simulink model "FEAD_TestRig"  (R2026a)
settings: Solver=ode23t  StartTime=0  StopTime=30  MaxStep=1e-3  RelTol=1e-4  AbsTol=1e-6
libraries: fl_lib x41, nesl_utility x27, simulink x1
settings Model: Creator=RICARDO  LastModifiedBy=RICARDO

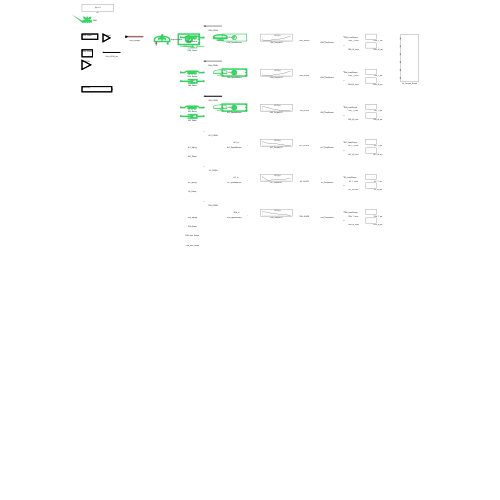
[thumbnail: Simulink's stored preview of the top-level diagram]
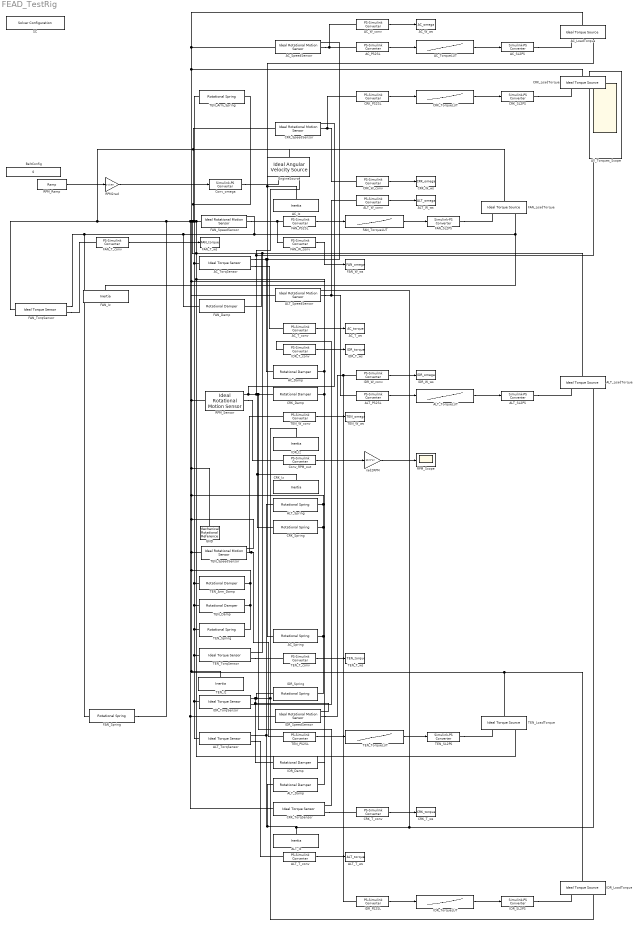
== system FEAD_TestRig ==
  AC_Damp : fl_lib/Mechanical/Rotational Elements/Rotational Damper  D=4.4060 N*m*s/rad  w_specify=off  w_priority=None  w=0 rad/s  w_nominal_specify=off  w_nominal_value=1  w_nominal_unit=rad/s  t_specify=off  t_priority=None  t=0 N*m  t_nominal_specify=off  t_nominal_value=1  t_nominal_unit=N*m
  AC_Iz : fl_lib/Mechanical/Rotational Elements/Inertia  inertia=0.005516 kg*m^2  num_ports=foundation.enum.numPorts2.one  w_specify=off  w_priority=High  w=0 rad/s  w_nominal_specify=off  w_nominal_value=1  w_nominal_unit=rad/s  t_specify=off  t_priority=None  t=0 N*m  t_nominal_specify=off  t_nominal_value=1  t_nominal_unit=N*m
  AC_LoadTorque : fl_lib/Mechanical/Mechanical Sources/Ideal Torque Source
  AC_PS2SL : nesl_utility/PS-Simulink Converter  PhysicalDomain=network_engine_domain  SubClassName=ps_output  LeftPortType=input  RightPortType=output  PseudoPeriodic=off  Frequencies=[]  VectorFormat=inherit  Unit=inherit  AffineConversion=off
  AC_SL2PS : nesl_utility/Simulink-PS Converter  PhysicalDomain=network_engine_domain  SubClassName=ps_input  LeftPortType=input  RightPortType=output  PseudoPeriodic=off  Frequencies=[]  NoiseDistribution=none  NoiseParameters=[]  Unit=1  AffineConversion=off  FilteringAndDerivatives=provide  SimscapeFilterOrder=1  InputFilterTimeConstant=0.001  UdotUserProvided=0
  AC_SpeedSensor : fl_lib/Mechanical/Mechanical Sensors/Ideal Rotational Motion Sensor  reference=foundation.enum.MeasurementReference.difference  acceleration_port=false  velocity_port=true  position_port=true  wrap_angle=false  offset=0 rad
  AC_Spring : fl_lib/Mechanical/Rotational Elements/Rotational Spring  spr_rate=4406.0 N*m/rad  w_specify=off  w_priority=None  w=0 rad/s  w_nominal_specify=off  w_nominal_value=1  w_nominal_unit=rad/s  t_specify=off  t_priority=None  t=0 N*m  t_nominal_specify=off  t_nominal_value=1  t_nominal_unit=N*m  phi_specify=off  phi_priority=High  phi=0 rad  phi_nominal_specify=off  phi_nominal_value=1  phi_nominal_unit=rad
  AC_T_conv : nesl_utility/PS-Simulink Converter  PhysicalDomain=network_engine_domain  SubClassName=ps_output  LeftPortType=input  RightPortType=output  PseudoPeriodic=off  Frequencies=[]  VectorFormat=inherit  Unit=inherit  AffineConversion=off
  AC_T_ws : ToWorkspace  VariableName=AC_torque  SampleTime=-1
  AC_TorqSensor : fl_lib/Mechanical/Mechanical Sensors/Ideal Torque Sensor
  AC_TorqueLUT : Lookup_n-D  NumberOfTableDimensions=1  BreakpointsForDimension1=[52.3599 83.7758 104.72 125.664 146.608 167.552 188.496 209.44]  Table=[19.0986 15.8757 16.5203 16.7113 16.5066 16.7113 17.4009 17.3797]  ExtrapMethod=Clip  InternalRulePriority=Speed  RndMeth=Simplest
  AC_W_conv : nesl_utility/PS-Simulink Converter  PhysicalDomain=network_engine_domain  SubClassName=ps_output  LeftPortType=input  RightPortType=output  PseudoPeriodic=off  Frequencies=[]  VectorFormat=inherit  Unit=inherit  AffineConversion=off
  AC_W_ws : ToWorkspace  VariableName=AC_omega  SampleTime=-1
  ALT_Damp : fl_lib/Mechanical/Rotational Elements/Rotational Damper  D=0.8823 N*m*s/rad  w_specify=off  w_priority=None  w=0 rad/s  w_nominal_specify=off  w_nominal_value=1  w_nominal_unit=rad/s  t_specify=off  t_priority=None  t=0 N*m  t_nominal_specify=off  t_nominal_value=1  t_nominal_unit=N*m
  ALT_Iz : fl_lib/Mechanical/Rotational Elements/Inertia  inertia=0.000543 kg*m^2  num_ports=foundation.enum.numPorts2.one  w_specify=off  w_priority=High  w=0 rad/s  w_nominal_specify=off  w_nominal_value=1  w_nominal_unit=rad/s  t_specify=off  t_priority=None  t=0 N*m  t_nominal_specify=off  t_nominal_value=1  t_nominal_unit=N*m
  ALT_LoadTorque : fl_lib/Mechanical/Mechanical Sources/Ideal Torque Source
  ALT_PS2SL : nesl_utility/PS-Simulink Converter  PhysicalDomain=network_engine_domain  SubClassName=ps_output  LeftPortType=input  RightPortType=output  PseudoPeriodic=off  Frequencies=[]  VectorFormat=inherit  Unit=inherit  AffineConversion=off
  ALT_SL2PS : nesl_utility/Simulink-PS Converter  PhysicalDomain=network_engine_domain  SubClassName=ps_input  LeftPortType=input  RightPortType=output  PseudoPeriodic=off  Frequencies=[]  NoiseDistribution=none  NoiseParameters=[]  Unit=1  AffineConversion=off  FilteringAndDerivatives=provide  SimscapeFilterOrder=1  InputFilterTimeConstant=0.001  UdotUserProvided=0
  ALT_SpeedSensor : fl_lib/Mechanical/Mechanical Sensors/Ideal Rotational Motion Sensor  reference=foundation.enum.MeasurementReference.difference  acceleration_port=false  velocity_port=true  position_port=true  wrap_angle=false  offset=0 rad
  ALT_Spring : fl_lib/Mechanical/Rotational Elements/Rotational Spring  spr_rate=882.3 N*m/rad  w_specify=off  w_priority=None  w=0 rad/s  w_nominal_specify=off  w_nominal_value=1  w_nominal_unit=rad/s  t_specify=off  t_priority=None  t=0 N*m  t_nominal_specify=off  t_nominal_value=1  t_nominal_unit=N*m  phi_specify=off  phi_priority=High  phi=0 rad  phi_nominal_specify=off  phi_nominal_value=1  phi_nominal_unit=rad
  ALT_T_conv : nesl_utility/PS-Simulink Converter  PhysicalDomain=network_engine_domain  SubClassName=ps_output  LeftPortType=input  RightPortType=output  PseudoPeriodic=off  Frequencies=[]  VectorFormat=inherit  Unit=inherit  AffineConversion=off
  ALT_T_ws : ToWorkspace  VariableName=ALT_torque  SampleTime=-1
  ALT_TorqSensor : fl_lib/Mechanical/Mechanical Sensors/Ideal Torque Sensor
  ALT_TorqueLUT : Lookup_n-D  NumberOfTableDimensions=1  BreakpointsForDimension1=[52.3599 83.7758 104.72 125.664 146.608 167.552 188.496 209.44]  Table=[30.5577 25.3056 25.4966 24.3507 22.0316 20.2923 18.8333 17.6662]  ExtrapMethod=Clip  InternalRulePriority=Speed  RndMeth=Simplest
  ALT_W_conv : nesl_utility/PS-Simulink Converter  PhysicalDomain=network_engine_domain  SubClassName=ps_output  LeftPortType=input  RightPortType=output  PseudoPeriodic=off  Frequencies=[]  VectorFormat=inherit  Unit=inherit  AffineConversion=off
  ALT_W_ws : ToWorkspace  VariableName=ALT_omega  SampleTime=-1
  All_Torques_Scope : Scope  NumInputPorts=6
  BeltConfig : Constant  Description=Belt: Gates MT620 AMD 8-Rib Aramid | L=1577mm | Ribs=8 | mu=0.35 | T_static=480N | EA=180000N  Value=0  OutDataTypeStr=double
  CRK_Damp : fl_lib/Mechanical/Rotational Elements/Rotational Damper  D=5.3358 N*m*s/rad  w_specify=off  w_priority=None  w=0 rad/s  w_nominal_specify=off  w_nominal_value=1  w_nominal_unit=rad/s  t_specify=off  t_priority=None  t=0 N*m  t_nominal_specify=off  t_nominal_value=1  t_nominal_unit=N*m
  CRK_Iz : fl_lib/Mechanical/Rotational Elements/Inertia  inertia=0.013296 kg*m^2  num_ports=foundation.enum.numPorts2.one  w_specify=off  w_priority=High  w=0 rad/s  w_nominal_specify=off  w_nominal_value=1  w_nominal_unit=rad/s  t_specify=off  t_priority=None  t=0 N*m  t_nominal_specify=off  t_nominal_value=1  t_nominal_unit=N*m
  CRK_LoadTorque : fl_lib/Mechanical/Mechanical Sources/Ideal Torque Source
  CRK_PS2SL : nesl_utility/PS-Simulink Converter  PhysicalDomain=network_engine_domain  SubClassName=ps_output  LeftPortType=input  RightPortType=output  PseudoPeriodic=off  Frequencies=[]  VectorFormat=inherit  Unit=inherit  AffineConversion=off
  CRK_SL2PS : nesl_utility/Simulink-PS Converter  PhysicalDomain=network_engine_domain  SubClassName=ps_input  LeftPortType=input  RightPortType=output  PseudoPeriodic=off  Frequencies=[]  NoiseDistribution=none  NoiseParameters=[]  Unit=1  AffineConversion=off  FilteringAndDerivatives=provide  SimscapeFilterOrder=1  InputFilterTimeConstant=0.001  UdotUserProvided=0
  CRK_SpeedSensor : fl_lib/Mechanical/Mechanical Sensors/Ideal Rotational Motion Sensor  reference=foundation.enum.MeasurementReference.difference  acceleration_port=false  velocity_port=true  position_port=true  wrap_angle=false  offset=0 rad
  CRK_Spring : fl_lib/Mechanical/Rotational Elements/Rotational Spring  spr_rate=5335.8 N*m/rad  w_specify=off  w_priority=None  w=0 rad/s  w_nominal_specify=off  w_nominal_value=1  w_nominal_unit=rad/s  t_specify=off  t_priority=None  t=0 N*m  t_nominal_specify=off  t_nominal_value=1  t_nominal_unit=N*m  phi_specify=off  phi_priority=High  phi=0 rad  phi_nominal_specify=off  phi_nominal_value=1  phi_nominal_unit=rad
  CRK_T_conv : nesl_utility/PS-Simulink Converter  PhysicalDomain=network_engine_domain  SubClassName=ps_output  LeftPortType=input  RightPortType=output  PseudoPeriodic=off  Frequencies=[]  VectorFormat=inherit  Unit=inherit  AffineConversion=off
  CRK_T_ws : ToWorkspace  VariableName=CRK_torque  SampleTime=-1
  CRK_TorqSensor : fl_lib/Mechanical/Mechanical Sensors/Ideal Torque Sensor
  CRK_TorqueLUT : Lookup_n-D  NumberOfTableDimensions=1  BreakpointsForDimension1=[52.3599 83.7758 104.72 125.664 146.608 167.552 188.496 209.44]  Table=[63.0254 54.3116 62.4524 66.5268 72.9157 78.7817 96.3948 106.188]  ExtrapMethod=Clip  InternalRulePriority=Speed  RndMeth=Simplest
  CRK_W_conv : nesl_utility/PS-Simulink Converter  PhysicalDomain=network_engine_domain  SubClassName=ps_output  LeftPortType=input  RightPortType=output  PseudoPeriodic=off  Frequencies=[]  VectorFormat=inherit  Unit=inherit  AffineConversion=off
  CRK_W_ws : ToWorkspace  VariableName=CRK_omega  SampleTime=-1
  Conv_RPM_out : nesl_utility/PS-Simulink Converter  PhysicalDomain=network_engine_domain  SubClassName=ps_output  LeftPortType=input  RightPortType=output  PseudoPeriodic=off  Frequencies=[]  VectorFormat=inherit  Unit=inherit  AffineConversion=off
  Conv_omega : nesl_utility/Simulink-PS Converter  PhysicalDomain=network_engine_domain  SubClassName=ps_input  LeftPortType=input  RightPortType=output  PseudoPeriodic=off  Frequencies=[]  NoiseDistribution=none  NoiseParameters=[]  Unit=1  AffineConversion=off  FilteringAndDerivatives=provide  SimscapeFilterOrder=1  InputFilterTimeConstant=0.001  UdotUserProvided=0
  EngineSource : fl_lib/Mechanical/Mechanical Sources/Ideal Angular Velocity Source
  FAN_Damp : fl_lib/Mechanical/Rotational Elements/Rotational Damper  D=5.0753 N*m*s/rad  w_specify=off  w_priority=None  w=0 rad/s  w_nominal_specify=off  w_nominal_value=1  w_nominal_unit=rad/s  t_specify=off  t_priority=None  t=0 N*m  t_nominal_specify=off  t_nominal_value=1  t_nominal_unit=N*m
  FAN_Iz : fl_lib/Mechanical/Rotational Elements/Inertia  inertia=0.015553 kg*m^2  num_ports=foundation.enum.numPorts2.one  w_specify=off  w_priority=High  w=0 rad/s  w_nominal_specify=off  w_nominal_value=1  w_nominal_unit=rad/s  t_specify=off  t_priority=None  t=0 N*m  t_nominal_specify=off  t_nominal_value=1  t_nominal_unit=N*m
  FAN_LoadTorque : fl_lib/Mechanical/Mechanical Sources/Ideal Torque Source
  FAN_PS2SL : nesl_utility/PS-Simulink Converter  PhysicalDomain=network_engine_domain  SubClassName=ps_output  LeftPortType=input  RightPortType=output  PseudoPeriodic=off  Frequencies=[]  VectorFormat=inherit  Unit=inherit  AffineConversion=off
  FAN_SL2PS : nesl_utility/Simulink-PS Converter  PhysicalDomain=network_engine_domain  SubClassName=ps_input  LeftPortType=input  RightPortType=output  PseudoPeriodic=off  Frequencies=[]  NoiseDistribution=none  NoiseParameters=[]  Unit=1  AffineConversion=off  FilteringAndDerivatives=provide  SimscapeFilterOrder=1  InputFilterTimeConstant=0.001  UdotUserProvided=0
  FAN_SpeedSensor : fl_lib/Mechanical/Mechanical Sensors/Ideal Rotational Motion Sensor  reference=foundation.enum.MeasurementReference.difference  acceleration_port=false  velocity_port=true  position_port=true  wrap_angle=false  offset=0 rad
  FAN_Spring : fl_lib/Mechanical/Rotational Elements/Rotational Spring  spr_rate=5075.3 N*m/rad  w_specify=off  w_priority=None  w=0 rad/s  w_nominal_specify=off  w_nominal_value=1  w_nominal_unit=rad/s  t_specify=off  t_priority=None  t=0 N*m  t_nominal_specify=off  t_nominal_value=1  t_nominal_unit=N*m  phi_specify=off  phi_priority=High  phi=0 rad  phi_nominal_specify=off  phi_nominal_value=1  phi_nominal_unit=rad
  FAN_T_conv : nesl_utility/PS-Simulink Converter  PhysicalDomain=network_engine_domain  SubClassName=ps_output  LeftPortType=input  RightPortType=output  PseudoPeriodic=off  Frequencies=[]  VectorFormat=inherit  Unit=inherit  AffineConversion=off
  FAN_T_ws : ToWorkspace  VariableName=FAN_torque  SampleTime=-1
  FAN_TorqSensor : fl_lib/Mechanical/Mechanical Sensors/Ideal Torque Sensor
  FAN_TorqueLUT : Lookup_n-D  NumberOfTableDimensions=1  BreakpointsForDimension1=[52.3599 83.7758 104.72 125.664 146.608 167.552 188.496 209.44]  Table=[9.5493 9.5493 17.1887 22.2817 31.3763 38.794 57.2958 68.2775]  ExtrapMethod=Clip  InternalRulePriority=Speed  RndMeth=Simplest
  FAN_W_conv : nesl_utility/PS-Simulink Converter  PhysicalDomain=network_engine_domain  SubClassName=ps_output  LeftPortType=input  RightPortType=output  PseudoPeriodic=off  Frequencies=[]  VectorFormat=inherit  Unit=inherit  AffineConversion=off
  FAN_W_ws : ToWorkspace  VariableName=FAN_omega  SampleTime=-1
  GND : fl_lib/Mechanical/Rotational Elements/Mechanical Rotational Reference
  IDR_Damp : fl_lib/Mechanical/Rotational Elements/Rotational Damper  D=1.4055 N*m*s/rad  w_specify=off  w_priority=None  w=0 rad/s  w_nominal_specify=off  w_nominal_value=1  w_nominal_unit=rad/s  t_specify=off  t_priority=None  t=0 N*m  t_nominal_specify=off  t_nominal_value=1  t_nominal_unit=N*m
  IDR_Iz : fl_lib/Mechanical/Rotational Elements/Inertia  inertia=0.000599 kg*m^2  num_ports=foundation.enum.numPorts2.one  w_specify=off  w_priority=High  w=0 rad/s  w_nominal_specify=off  w_nominal_value=1  w_nominal_unit=rad/s  t_specify=off  t_priority=None  t=0 N*m  t_nominal_specify=off  t_nominal_value=1  t_nominal_unit=N*m
  IDR_LoadTorque : fl_lib/Mechanical/Mechanical Sources/Ideal Torque Source
  IDR_PS2SL : nesl_utility/PS-Simulink Converter  PhysicalDomain=network_engine_domain  SubClassName=ps_output  LeftPortType=input  RightPortType=output  PseudoPeriodic=off  Frequencies=[]  VectorFormat=inherit  Unit=inherit  AffineConversion=off
  IDR_SL2PS : nesl_utility/Simulink-PS Converter  PhysicalDomain=network_engine_domain  SubClassName=ps_input  LeftPortType=input  RightPortType=output  PseudoPeriodic=off  Frequencies=[]  NoiseDistribution=none  NoiseParameters=[]  Unit=1  AffineConversion=off  FilteringAndDerivatives=provide  SimscapeFilterOrder=1  InputFilterTimeConstant=0.001  UdotUserProvided=0
  IDR_SpeedSensor : fl_lib/Mechanical/Mechanical Sensors/Ideal Rotational Motion Sensor  reference=foundation.enum.MeasurementReference.difference  acceleration_port=false  velocity_port=true  position_port=true  wrap_angle=false  offset=0 rad
  IDR_Spring : fl_lib/Mechanical/Rotational Elements/Rotational Spring  spr_rate=1405.5 N*m/rad  w_specify=off  w_priority=None  w=0 rad/s  w_nominal_specify=off  w_nominal_value=1  w_nominal_unit=rad/s  t_specify=off  t_priority=None  t=0 N*m  t_nominal_specify=off  t_nominal_value=1  t_nominal_unit=N*m  phi_specify=off  phi_priority=High  phi=0 rad  phi_nominal_specify=off  phi_nominal_value=1  phi_nominal_unit=rad
  IDR_T_conv : nesl_utility/PS-Simulink Converter  PhysicalDomain=network_engine_domain  SubClassName=ps_output  LeftPortType=input  RightPortType=output  PseudoPeriodic=off  Frequencies=[]  VectorFormat=inherit  Unit=inherit  AffineConversion=off
  IDR_T_ws : ToWorkspace  VariableName=IDR_torque  SampleTime=-1
  IDR_TorqSensor : fl_lib/Mechanical/Mechanical Sensors/Ideal Torque Sensor
  IDR_TorqueLUT : Lookup_n-D  NumberOfTableDimensions=1  BreakpointsForDimension1=[52.3599 83.7758 104.72 125.664 146.608 167.552 188.496 209.44]  Table=[1.90986 1.79049 1.62338 1.59155 1.5006 1.49208 1.43239 1.43239]  ExtrapMethod=Clip  InternalRulePriority=Speed  RndMeth=Simplest
  IDR_W_conv : nesl_utility/PS-Simulink Converter  PhysicalDomain=network_engine_domain  SubClassName=ps_output  LeftPortType=input  RightPortType=output  PseudoPeriodic=off  Frequencies=[]  VectorFormat=inherit  Unit=inherit  AffineConversion=off
  IDR_W_ws : ToWorkspace  VariableName=IDR_omega  SampleTime=-1
  RPM2rad : Gain  Gain=2*pi/60
  RPM_Ramp : simulink/Sources/Ramp  slope=(2000-600)/15  start=0  InitialOutput=600
  RPM_Scope : Scope
  RPM_Sensor : fl_lib/Mechanical/Mechanical Sensors/Ideal Rotational Motion Sensor  reference=foundation.enum.MeasurementReference.difference  acceleration_port=false  velocity_port=true  position_port=true  wrap_angle=false  offset=0 rad
  SC : nesl_utility/Solver Configuration  PhysicalDomain=network_engine_domain  SubClassName=solver  LeftPortType=input  RightPortType=generic  Tones=[]  Harmonics=[]  SimulateNoise=off  Profile=off  UseLocalSampling=off  EnableSwitchedLinearOptims=on  FrequencyDomain=off  UseCCode=off  RelTol=0.001  AbsTol=0.001  MinStep=1e-09  ToWorkspace=off  RevertToSquareIcSolve=off  NumHomotopyIterations=100  PhasorMode=off  PhasorModeNumHarmonics=1  ConsistencySolver=NEWTON_XTOL_AFTER_FTOL  CanonicalOrdering=CANONICAL  OptimizeIntermediates=OPTIMIZED  IndexReductionMethod=DerivativeReplacement  DoDC=off  ResidualTolerance=1e-09  ConsistencyTolSource=GLOBAL  ConsistencyAbsTol=0.001  ConsistencyRelTol=0.001  ConsistencyTolFactor=0.001  UseLocalSolver=off  LocalSolverChoice=NE_BACKWARD_EULER_ADVANCER  ResolveIndetEquations=on  FunctionEvalNumThread=1  LocalSolverSampleTime=0.001  DoFixedCost=off  MaxNonlinIter=3  MaxModeIter=2  ComputeImpulses=off  ImpulseIterations=2  LinearAlgebra=auto  LinearAlgebraNumThread=0  EquationFormulation=NE_TIME_EF  DelaysMemoryBudget=1024  AutomaticFiltering=on  FilteringTimeConstant=0.001  PartitionStorageMethod=AS_NEEDED  PartitionMemoryBudget=1024  PartitionMethod=ROBUST  MultibodyUseLocalSolver=off  MultibodyLocalSolverChoice=ODE1  MultibodyLocalSolverSampleTime=0.001
  TEN_Arm_Damp : fl_lib/Mechanical/Rotational Elements/Rotational Damper  D=0.08830 N*m*s/rad  w_specify=off  w_priority=None  w=0 rad/s  w_nominal_specify=off  w_nominal_value=1  w_nominal_unit=rad/s  t_specify=off  t_priority=None  t=0 N*m  t_nominal_specify=off  t_nominal_value=1  t_nominal_unit=N*m
  TEN_Arm_Spring : fl_lib/Mechanical/Rotational Elements/Rotational Spring  spr_rate=0.8830 N*m/rad  w_specify=off  w_priority=None  w=0 rad/s  w_nominal_specify=off  w_nominal_value=1  w_nominal_unit=rad/s  t_specify=off  t_priority=None  t=0 N*m  t_nominal_specify=off  t_nominal_value=1  t_nominal_unit=N*m  phi_specify=off  phi_priority=High  phi=0 rad  phi_nominal_specify=off  phi_nominal_value=1  phi_nominal_unit=rad
  TEN_Damp : fl_lib/Mechanical/Rotational Elements/Rotational Damper  D=1.4908 N*m*s/rad  w_specify=off  w_priority=None  w=0 rad/s  w_nominal_specify=off  w_nominal_value=1  w_nominal_unit=rad/s  t_specify=off  t_priority=None  t=0 N*m  t_nominal_specify=off  t_nominal_value=1  t_nominal_unit=N*m
  TEN_Iz : fl_lib/Mechanical/Rotational Elements/Inertia  inertia=0.000674 kg*m^2  num_ports=foundation.enum.numPorts2.one  w_specify=off  w_priority=High  w=0 rad/s  w_nominal_specify=off  w_nominal_value=1  w_nominal_unit=rad/s  t_specify=off  t_priority=None  t=0 N*m  t_nominal_specify=off  t_nominal_value=1  t_nominal_unit=N*m
  TEN_LoadTorque : fl_lib/Mechanical/Mechanical Sources/Ideal Torque Source
  TEN_PS2SL : nesl_utility/PS-Simulink Converter  PhysicalDomain=network_engine_domain  SubClassName=ps_output  LeftPortType=input  RightPortType=output  PseudoPeriodic=off  Frequencies=[]  VectorFormat=inherit  Unit=inherit  AffineConversion=off
  TEN_SL2PS : nesl_utility/Simulink-PS Converter  PhysicalDomain=network_engine_domain  SubClassName=ps_input  LeftPortType=input  RightPortType=output  PseudoPeriodic=off  Frequencies=[]  NoiseDistribution=none  NoiseParameters=[]  Unit=1  AffineConversion=off  FilteringAndDerivatives=provide  SimscapeFilterOrder=1  InputFilterTimeConstant=0.001  UdotUserProvided=0
  TEN_SpeedSensor : fl_lib/Mechanical/Mechanical Sensors/Ideal Rotational Motion Sensor  reference=foundation.enum.MeasurementReference.difference  acceleration_port=false  velocity_port=true  position_port=true  wrap_angle=false  offset=0 rad
  TEN_Spring : fl_lib/Mechanical/Rotational Elements/Rotational Spring  spr_rate=1490.8 N*m/rad  w_specify=off  w_priority=None  w=0 rad/s  w_nominal_specify=off  w_nominal_value=1  w_nominal_unit=rad/s  t_specify=off  t_priority=None  t=0 N*m  t_nominal_specify=off  t_nominal_value=1  t_nominal_unit=N*m  phi_specify=off  phi_priority=High  phi=0 rad  phi_nominal_specify=off  phi_nominal_value=1  phi_nominal_unit=rad
  TEN_T_conv : nesl_utility/PS-Simulink Converter  PhysicalDomain=network_engine_domain  SubClassName=ps_output  LeftPortType=input  RightPortType=output  PseudoPeriodic=off  Frequencies=[]  VectorFormat=inherit  Unit=inherit  AffineConversion=off
  TEN_T_ws : ToWorkspace  VariableName=TEN_torque  SampleTime=-1
  TEN_TorqSensor : fl_lib/Mechanical/Mechanical Sensors/Ideal Torque Sensor
  TEN_TorqueLUT : Lookup_n-D  NumberOfTableDimensions=1  BreakpointsForDimension1=[52.3599 83.7758 104.72 125.664 146.608 167.552 188.496 209.44]  Table=[1.90986 1.79049 1.62338 1.59155 1.5006 1.49208 1.43239 1.28916]  ExtrapMethod=Clip  InternalRulePriority=Speed  RndMeth=Simplest
  TEN_W_conv : nesl_utility/PS-Simulink Converter  PhysicalDomain=network_engine_domain  SubClassName=ps_output  LeftPortType=input  RightPortType=output  PseudoPeriodic=off  Frequencies=[]  VectorFormat=inherit  Unit=inherit  AffineConversion=off
  TEN_W_ws : ToWorkspace  VariableName=TEN_omega  SampleTime=-1
  rad2RPM : Gain  Gain=60/(2*pi)
  wires:
  RPM_Ramp/1 -> RPM2rad/1
  IDR_TorqueLUT/1 -> IDR_SL2PS/1
  AC_W_conv/1 -> AC_W_ws/1
  RPM2rad/1 -> Conv_omega/1
  FAN_T_conv/1 -> FAN_T_ws/1
  ALT_T_conv/1 -> ALT_T_ws/1
  FAN_W_conv/1 -> FAN_W_ws/1
  TEN_TorqueLUT/1 -> TEN_SL2PS/1
  IDR_T_conv/1 -> IDR_T_ws/1
  CRK_W_conv/1 -> CRK_W_ws/1
  FAN_PS2SL/1 -> FAN_TorqueLUT/1
  AC_T_conv/1 -> AC_T_ws/1
  TEN_W_conv/1 -> TEN_W_ws/1
  Conv_RPM_out/1 -> rad2RPM/1
  TEN_T_conv/1 -> TEN_T_ws/1
  TEN_PS2SL/1 -> TEN_TorqueLUT/1
  AC_PS2SL/1 -> AC_TorqueLUT/1
  CRK_PS2SL/1 -> CRK_TorqueLUT/1
  FAN_TorqueLUT/1 -> FAN_SL2PS/1
  ALT_W_conv/1 -> ALT_W_ws/1
  CRK_TorqueLUT/1 -> CRK_SL2PS/1
  IDR_W_conv/1 -> IDR_W_ws/1
  ALT_PS2SL/1 -> ALT_TorqueLUT/1
  ALT_TorqueLUT/1 -> ALT_SL2PS/1
  rad2RPM/1 -> RPM_Scope/1
  CRK_T_conv/1 -> CRK_T_ws/1
  IDR_PS2SL/1 -> IDR_TorqueLUT/1
  AC_TorqueLUT/1 -> AC_SL2PS/1
  connections:
  FAN_SpeedSensor/RConn2 -- FAN_PS2SL/LConn1 -- FAN_W_conv/LConn1
  FAN_TorqSensor/RConn1 -- FAN_LoadTorque/RConn2 -- FAN_Iz/LConn1 -- FAN_SpeedSensor/RConn1 -- FAN_Damp/LConn1 -- FAN_Spring/LConn1
  FAN_TorqSensor/RConn2 -- FAN_T_conv/LConn1
  Conv_omega/RConn1 -- EngineSource/RConn1
  FAN_Spring/RConn1 -- FAN_TorqSensor/LConn1 -- EngineSource/LConn1 -- IDR_SpeedSensor/LConn1 -- CRK_TorqSensor/LConn1 -- TEN_LoadTorque/LConn1 -- IDR_LoadTorque/LConn1 -- TEN_Iz/LConn1 -- TEN_Spring/RConn1 -- TEN_Damp/RConn1 -- TEN_Arm_Damp/RConn1 -- TEN_SpeedSensor/LConn1 -- TEN_SpeedSensor/RConn1 -- AC_Spring/RConn1 -- IDR_Spring/RConn1 -- CRK_Spring/RConn1 -- ALT_Spring/RConn1 -- GND/LConn1 -- RPM_Sensor/LConn1 -- IDR_Damp/RConn1 -- CRK_Damp/RConn1 -- AC_Damp/RConn1 -- ALT_SpeedSensor/LConn1 -- AC_SpeedSensor/LConn1 -- AC_LoadTorque/LConn1 -- CRK_LoadTorque/LConn1 -- ALT_LoadTorque/LConn1 -- TEN_TorqSensor/RConn1 -- CRK_SpeedSensor/LConn1 -- FAN_LoadTorque/LConn1 -- TEN_Arm_Spring/RConn1 -- ALT_TorqSensor/LConn1 -- IDR_TorqSensor/LConn1 -- TEN_TorqSensor/LConn1 -- TEN_Spring/LConn1 -- TEN_Damp/LConn1 -- TEN_Arm_Damp/LConn1 -- AC_TorqSensor/LConn1 -- TEN_LoadTorque/RConn2 -- ALT_Damp/RConn1 -- FAN_Damp/RConn1 -- FAN_SpeedSensor/LConn1 -- TEN_Arm_Spring/LConn1
  RPM_Sensor/RConn1 -- CRK_Spring/LConn1 -- CRK_Iz/LConn1 -- CRK_TorqSensor/RConn1 -- CRK_Damp/LConn1 -- EngineSource/RConn2 -- CRK_LoadTorque/RConn2 -- CRK_SpeedSensor/RConn1
  AC_TorqSensor/RConn2 -- AC_T_conv/LConn1
  AC_TorqSensor/RConn1 -- AC_Spring/LConn1 -- AC_SpeedSensor/RConn1 -- AC_LoadTorque/RConn2 -- AC_Iz/LConn1 -- AC_Damp/LConn1
  RPM_Sensor/RConn2 -- Conv_RPM_out/LConn1
  TEN_SpeedSensor/RConn2 -- TEN_PS2SL/LConn1 -- TEN_W_conv/LConn1
  TEN_TorqSensor/RConn2 -- TEN_T_conv/LConn1
  IDR_TorqSensor/RConn2 -- IDR_T_conv/LConn1
  IDR_TorqSensor/RConn1 -- IDR_SpeedSensor/RConn1 -- IDR_Damp/LConn1 -- IDR_LoadTorque/RConn2 -- IDR_Iz/LConn1 -- IDR_Spring/LConn1
  ALT_TorqSensor/RConn2 -- ALT_T_conv/LConn1
  ALT_TorqSensor/RConn1 -- ALT_LoadTorque/RConn2 -- ALT_SpeedSensor/RConn1 -- ALT_Iz/LConn1 -- ALT_Damp/LConn1 -- ALT_Spring/LConn1
  AC_SpeedSensor/RConn2 -- AC_PS2SL/LConn1 -- AC_W_conv/LConn1
  CRK_SpeedSensor/RConn2 -- CRK_PS2SL/LConn1 -- CRK_W_conv/LConn1
  ALT_SpeedSensor/RConn2 -- ALT_PS2SL/LConn1 -- ALT_W_conv/LConn1
  CRK_TorqSensor/RConn2 -- CRK_T_conv/LConn1
  IDR_SpeedSensor/RConn2 -- IDR_W_conv/LConn1 -- IDR_PS2SL/LConn1
  IDR_SL2PS/RConn1 -- IDR_LoadTorque/RConn1
  ALT_SL2PS/RConn1 -- ALT_LoadTorque/RConn1
  CRK_SL2PS/RConn1 -- CRK_LoadTorque/RConn1
  TEN_SL2PS/RConn1 -- TEN_LoadTorque/RConn1
  FAN_SL2PS/RConn1 -- FAN_LoadTorque/RConn1
  AC_SL2PS/RConn1 -- AC_LoadTorque/RConn1
